simulink model "x1_myfoc_transform"  (R2025b)
settings: Solver=ode23t  StartTime=0.0  StopTime=0.5  RelTol=1e-3
values from neighbouring files (symbols this model uses):
  Ts = 1/SwitchFrequency    (= 5e-05)    [foc_para.m]
undefined symbols (not defined in the file or in its folder): DiscIntNeverNeededParam
settings Model: Creator=disnox  LastModifiedBy=yolo
settings DataIOCC: ReturnWorkspaceOutputs=off
settings DebuggingCC: SaveWithParameterizedLinksMsg=none  ParameterPrecisionLossMsg=none
settings HardwareCC: ProdBitPerPointer=32.0  ProdBitPerSizeT=32.0  ProdBitPerPtrDiffT=32.0  ProdLargestAtomicInteger=Long  ProdLargestAtomicFloat=Double  ProdWordSize=32.0  ProdHWDeviceType=ARM Compatible->ARM Cortex-M
settings RTWCC: GPUComputeCapability=3.5

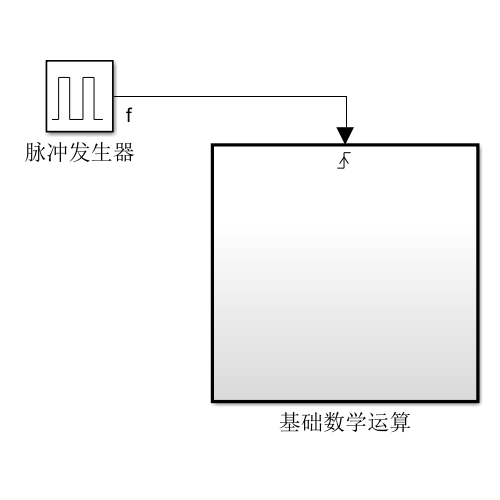
[thumbnail: Simulink's stored preview of the top-level diagram]
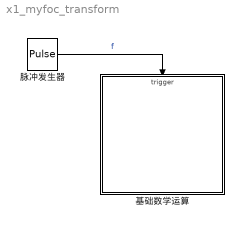
== system x1_myfoc_transform ==
  基础数学运算 : Subsystem
  脉冲发生器 : DiscretePulseGenerator  PulseType=Time based  Period=Ts  PulseWidth=5
  wires:
  脉冲发生器/1 -> 基础数学运算/Trigger  "f"

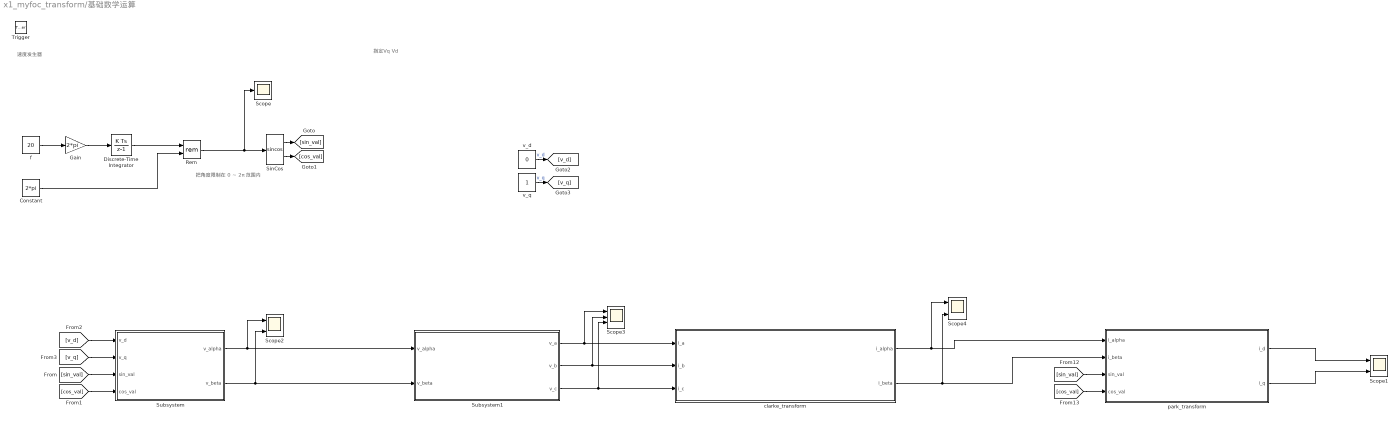
== system x1_myfoc_transform/基础数学运算 ==
  note: 指定Vq Vd
  note: 把角度限制在 0 ~ 2π 范围内
  note: 速度发生器
  Trigger : TriggerPort  VariantControl=(inherit)  PortDimensions=1
  Constant : Constant  Value=2*pi
  Discrete-Time Integrator : DiscreteIntegrator  SampleTime=-1  ICPrevOutput=DiscIntNeverNeededParam  ICPrevScaledInput=DiscIntNeverNeededParam
  Gain : Gain  Gain=2*pi
  Rem : Math  Operator=rem
  Scope : Scope
      settings: ActiveDisplayYMinimum=4.21833  ActiveDisplayYMaximum=5.47784  DataLoggingVariableName=ScopeData4
  Scope1 : Scope  NumInputPorts=2
      settings: ActiveDisplayYMinimum=-0.125  ActiveDisplayYMaximum=1.125  DataLoggingVariableName=ScopeData6
  Scope2 : Scope  NumInputPorts=2
      settings: ActiveDisplayYMinimum=-0.125  ActiveDisplayYMaximum=1.125
  Scope3 : Scope  NumInputPorts=3
      settings: ActiveDisplayYMinimum=-0.125  ActiveDisplayYMaximum=1.125
  Scope4 : Scope  NumInputPorts=2
      settings: ActiveDisplayYMinimum=-0.125  ActiveDisplayYMaximum=1.125  DataLoggingVariableName=ScopeData2
  SinCos : Trigonometry  Operator=sincos
  Subsystem : Subsystem
  Subsystem1 : Subsystem
  clarke_transform : Subsystem  TreatAsAtomicUnit=on
      settings: RTWSystemCode=Nonreusable function  RTWFcnNameOpts=Use subsystem name
  f : Constant  Value=20
  park_transform : Subsystem  TreatAsAtomicUnit=on
      settings: RTWSystemCode=Nonreusable function  RTWFcnNameOpts=Use subsystem name
  v_d : Constant  Value=0
  v_q : Constant
  wires:
  SinCos/2 -> [cos_val]
  Constant/1 -> Rem/2
  Gain/1 -> Discrete-Time Integrator/1
  f/1 -> Gain/1
  SinCos/1 -> [sin_val]
  Discrete-Time Integrator/1 -> Rem/1
  Rem/1 -> SinCos/1, Scope/1
  v_d/1 -> [v_d]  "v_d"
  v_q/1 -> [v_q]  "v_q"
  [v_d] -> Subsystem/1(v_d)
  [v_q] -> Subsystem/2(v_q)
  [sin_val] -> Subsystem/3(sin_val)
  [cos_val] -> Subsystem/4(cos_val)
  Subsystem/1(v_alpha) -> Scope2/1, Subsystem1/1(v_alpha)
  Subsystem/2(v_beta) -> Scope2/2, Subsystem1/2(v_beta)
  Subsystem1/1(v_a) -> Scope3/1, clarke_transform/1(i_a)
  Subsystem1/2(v_b) -> Scope3/2, clarke_transform/2(i_b)
  Subsystem1/3(v_c) -> Scope3/3, clarke_transform/3(i_c)
  park_transform/1(i_d) -> Scope1/1
  [cos_val] -> park_transform/4(cos_val)
  park_transform/2(i_q) -> Scope1/2
  [sin_val] -> park_transform/3(sin_val)
  clarke_transform/1(i_alpha) -> Scope4/1, park_transform/1(i_alpha)
  clarke_transform/2(i_beta) -> Scope4/2, park_transform/2(i_beta)

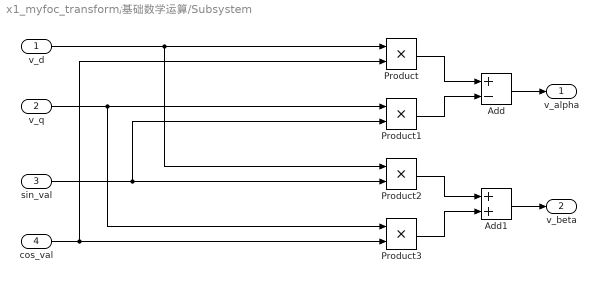
== system x1_myfoc_transform/基础数学运算/Subsystem ==
  v_d : Inport
  v_q : Inport  Port=2
  sin_val : Inport  Port=3
  cos_val : Inport  Port=4
  Add : Sum  Inputs=+-
  Add1 : Sum  AccumDataTypeStr=double
  Product{,1..3} (4 alike) : Product
  v_alpha : Outport
  v_beta : Outport  Port=2
  wires:
  Add1/1 -> v_beta/1
  v_q/1 -> Product1/1, Product3/1
  Add/1 -> v_alpha/1
  Product/1 -> Add/1
  Product1/1 -> Add/2
  Product2/1 -> Add1/1
  sin_val/1 -> Product2/2, Product1/2
  v_d/1 -> Product2/1, Product/1
  Product3/1 -> Add1/2
  cos_val/1 -> Product3/2, Product/2

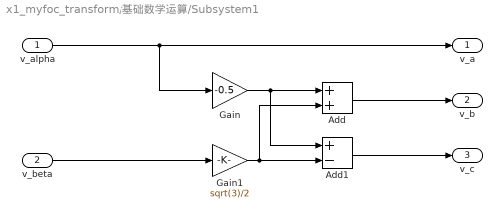
== system x1_myfoc_transform/基础数学运算/Subsystem1 ==
  v_alpha : Inport
  v_beta : Inport  Port=2
  Add : Sum
  Add1 : Sum  Inputs=+-
  Gain : Gain  Gain=-0.5
  Gain1 : Gain  Gain=sqrt(3)/2
  v_a : Outport
  v_b : Outport  Port=2
  v_c : Outport  Port=3
  wires:
  Gain/1 -> Add1/1, Add/1
  Add1/1 -> v_c/1
  Add/1 -> v_b/1
  Gain1/1 -> Add/2, Add1/2
  v_alpha/1 -> Gain/1, v_a/1
  v_beta/1 -> Gain1/1

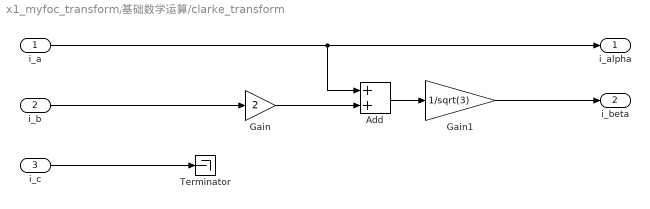
== system x1_myfoc_transform/基础数学运算/clarke_transform ==
  i_a : Inport
  i_b : Inport  Port=2
  i_c : Inport  Port=3
  Add : Sum
  Gain : Gain  Gain=2
  Gain1 : Gain  Gain=1/sqrt(3)
  Terminator : Terminator
  i_alpha : Outport
  i_beta : Outport  Port=2
  wires:
  i_a/1 -> Add/1, i_alpha/1
  i_b/1 -> Gain/1
  Gain/1 -> Add/2
  Add/1 -> Gain1/1
  Gain1/1 -> i_beta/1
  i_c/1 -> Terminator/1

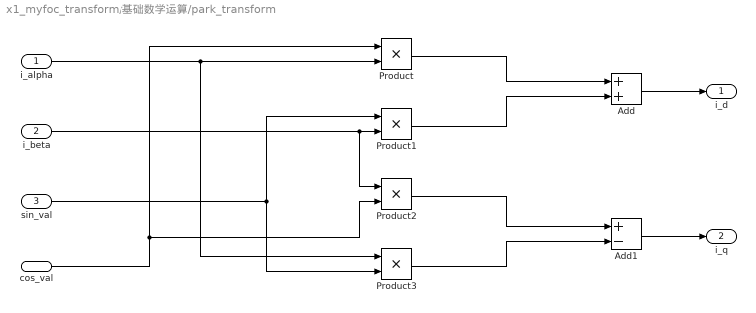
== system x1_myfoc_transform/基础数学运算/park_transform ==
  i_alpha : Inport
  i_beta : Inport  Port=2
  sin_val : Inport  Port=3
  cos_val : Inport  Port=4
  Add : Sum
  Add1 : Sum  Inputs=+-
  Product{,1..3} (4 alike) : Product
  i_d : Outport
  i_q : Outport  Port=2
  wires:
  i_alpha/1 -> Product/2, Product3/1
  cos_val/1 -> Product2/2, Product/1
  sin_val/1 -> Product3/2, Product1/1
  i_beta/1 -> Product2/1, Product1/2
  Product/1 -> Add/1
  Product1/1 -> Add/2
  Add/1 -> i_d/1
  Product2/1 -> Add1/1
  Product3/1 -> Add1/2
  Add1/1 -> i_q/1
